simulink model "feedback_boost"  (R2022b)
settings: Solver=FixedStepAuto  StartTime=0.0  StopTime=2  FixedStep=1e-6  RelTol=1e-3
undefined symbols (not defined in the file): poremecaj, promena_ref, R, ref_V, sigma, vg, wpref
libraries: cstblocks x1
settings Model: SimulationMode=accelerator  Creator=user  LastModifiedBy=user

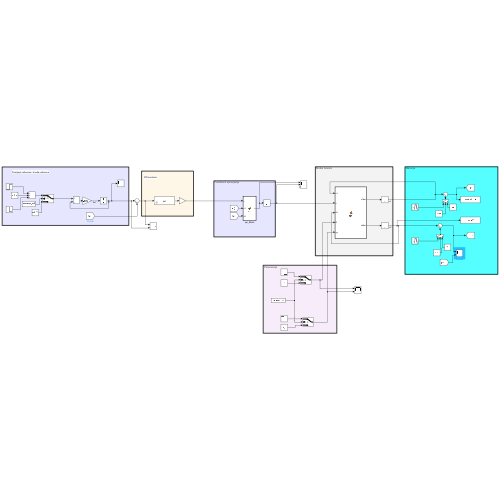
[thumbnail: Simulink's stored preview of the top-level diagram]
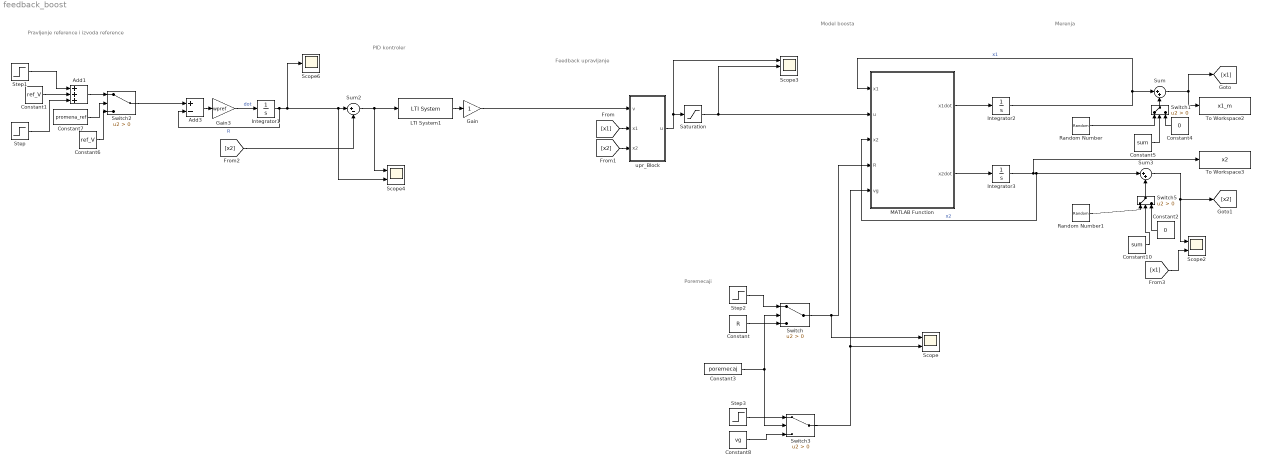
== system feedback_boost ==
  note: Merenja
  note: Model boosta
  note: Poremecaji
  note: Feedback upravljanje
  note: PID kontroler
  note: Pravljenje reference i izvoda reference
  Add1 : Sum  Inputs=+++
  Add3 : Sum  Inputs=+-
  Constant : Constant  Value=R
  Constant1 : Constant  Value=ref_V  SampleTime=-1
  Constant10 : Constant  Value=sum
  Constant2 : Constant  Value=0
  Constant3 : Constant  Value=poremecaj
  Constant4 : Constant  Value=0
  Constant5 : Constant  Value=sum
  Constant6 : Constant  Value=ref_V  SampleTime=-1
  Constant7 : Constant  Value=promena_ref
  Constant8 : Constant  Value=vg  SampleTime=0
  Gain : Gain
  Gain3 : Gain  Gain=wpref
  Integrator1 : Integrator  InitialCondition=12
  Integrator2 : Integrator  InitialCondition=3.5
  Integrator3 : Integrator  InitialCondition=18
  LTI System1 : cstblocks/LTI System  sys=pid  IC=[]
  MATLAB Function : MATLAB Function  TreatAsAtomicUnit=on
  Random Number : RandomNumber  Variance=sigma^2  SampleTime=0.01
  Random Number1 : RandomNumber  Variance=sigma^2  Seed=2043  SampleTime=0.01
  Saturation : Saturate  UpperLimit=1  LowerLimit=0
  Scope : Scope  NumInputPorts=2
  Scope2 : Scope  NumInputPorts=2
  Scope3 : Scope  NumInputPorts=3
  Scope4 : Scope  NumInputPorts=2
  Scope6 : Scope
  Step : Step  Time=1.5  After=-2
  Step1 : Step  Time=1.1  SampleTime=0
  Step2 : Step  Time=0.9  Before=R  After=0.9*R  SampleTime=0
  Step3 : Step  Time=0.5  Before=vg  After=vg-1  SampleTime=0
  Sum : Sum  Inputs=|++
  Sum2 : Sum  Inputs=|+-
  Sum3 : Sum  Inputs=|++
  Switch{,1..3,5} (5 alike) : Switch  Criteria=u2 > Threshold  SaturateOnIntegerOverflow=off  InputSameDT=off
  To Workspace2 : ToWorkspace  VariableName=x1_m  SampleTime=1e-5
      settings: Save2DSignal=2-D array (concatenate along first dimension)
  To Workspace3 : ToWorkspace  VariableName=x2  SampleTime=1e-5
      settings: Save2DSignal=2-D array (concatenate along first dimension)
  upr_Block : MATLAB Function  TreatAsAtomicUnit=on
  wires:
  Integrator1/1 -> Add3/2, Scope6/1, Scope4/2, Sum2/1  "R"
  Switch2/1 -> Add3/1
  Constant7/1 -> Switch2/2
  Add3/1 -> Gain3/1
  Add1/1 -> Switch2/1
  Gain3/1 -> Integrator1/1  "dot"
  Step1/1 -> Add1/1
  Constant6/1 -> Switch2/3
  Constant1/1 -> Add1/2
  Step/1 -> Add1/3
  [x2] -> upr_Block/3(x2)
  Gain/1 -> upr_Block/1(v)
  [x1] -> upr_Block/2(x1)
  Sum2/1 -> LTI System1/1, Scope4/1
  upr_Block/1(u) -> Scope3/1, Saturation/1
  Sum3/1 -> [x2], Scope2/1
  Integrator3/1 -> MATLAB Function/3(x2), Sum3/1, To Workspace3/1  "x2"
  Random Number1/1 -> Switch5/1
  Switch5/1 -> Sum3/2
  Constant2/1 -> Switch5/3
  Constant10/1 -> Switch5/2
  [x1] -> Scope2/2
  Constant5/1 -> Switch1/2
  Constant4/1 -> Switch1/3
  Switch1/1 -> Sum/2
  Random Number/1 -> Switch1/1
  Sum/1 -> [x1], To Workspace2/1
  Integrator2/1 -> Sum/1, MATLAB Function/1(x1)  "x1"
  MATLAB Function/2(x2dot) -> Integrator3/1
  MATLAB Function/1(x1dot) -> Integrator2/1
  Step3/1 -> Switch3/1
  Constant8/1 -> Switch3/3
  Switch3/1 -> Scope/2, MATLAB Function/5(vg)
  Constant3/1 -> Switch3/2, Switch/2
  Step2/1 -> Switch/1
  Constant/1 -> Switch/3
  Switch/1 -> Scope/1, MATLAB Function/4(R)
  [x2] -> Sum2/2
  LTI System1/1 -> Gain/1
  Saturation/1 -> MATLAB Function/2(u), Scope3/2

== matlab function feedback_boost/upr_Block ==
  data: v input; u output; x1 input; x2 input
function u  = fcn(v,x1,x2)
u = -(v/2000-x1+x2/15)/x1;

end

== matlab function feedback_boost/MATLAB Function ==
  data: x1 input; u input; x1dot output; x2 input; x2dot output; R input; vg input
function [x1dot,x2dot] = fcn(x1,u,x2,R,vg)
L=250e-6;   % H
vd=0.7;     % V
Rd=0.5;     % Ohm
Rl=0.2;     % Ohm
C=500e-6;   % F
Ron=0.3;      % Ohm

% L=250e-6;   % H
% vd=0.0;     % V
% Rd=0.0;     % Ohm
% Rl=0.0;     % Ohm
% C=500e-6;   % F
% Ron=0.0;      % Ohm


x1dot =  u*(x1*((Rd + Rl)/L - (Rl + Ron)/L) + x2/L - vd/L) - x2/L - vd/L + vg/L - (x1*(Rd + Rl))/L;
x2dot= x1/C-x2/R/C+(-x1)/C*u;
